simulink model "ame532Project1_GimbalDynamicsModel_2022b"  (R2022b)
settings: Solver=ode4  StartTime=0.0  StopTime=10  FixedStep=0.01  RelTol=1e-3
model workspace (MAT data in the model file):
  theta : Simulink.Parameter (value not decoded)
values from neighbouring files (symbols this model uses):
  a0_s2 = 0    [AeroData.m]
  a0_s3 = 0    [AeroData.m]
  a0_s4 = 0.05    [AeroData.m]
  a0_s5 = 0.05    [AeroData.m]
  CD0_s2 = 0.01    [AeroData.m]
  CD0_s3 = 0.01    [AeroData.m]
  CD0_s4 = 0.01    [AeroData.m]
  CD0_s5 = 0.01    [AeroData.m]
  CDa_s2 = 1    [AeroData.m]
  CDa_s3 = 1    [AeroData.m]
  CDa_s4 = 1    [AeroData.m]
  CDa_s5 = 1    [AeroData.m]
  CL0_s2 = 0    [AeroData.m]
  CL0_s3 = 0    [AeroData.m]
  CL0_s4 = 0.05    [AeroData.m]
  CL0_s5 = 0.05    [AeroData.m]
  CM0_s2 = 0    [AeroData.m]
  CM0_s3 = 0    [AeroData.m]
  CM0_s4 = -0.05    [AeroData.m]
  CM0_s5 = -0.05    [AeroData.m]
  CMa_s2 = 0    [AeroData.m]
  CMa_s3 = 0    [AeroData.m]
  CMa_s4 = 0    [AeroData.m]
  CMa_s5 = 0    [AeroData.m]
  e_s2 = 0.8    [AeroData.m]
  e_s3 = 0.8    [AeroData.m]
  e_s4 = 0.9    [AeroData.m]
  e_s5 = 0.9    [AeroData.m]
  i_s2 = 0    [AeroData.m]
  i_s3 = 0    [AeroData.m]
  i_s4 = 0.05    [AeroData.m]
  i_s5 = 0.05    [AeroData.m]
  Jxx = 1    [Sim_sixDOFdriverScript.m]
  Jxy = 0.    (= 0)    [Sim_sixDOFdriverScript.m]
  Jxz = 3    [Sim_sixDOFdriverScript.m]
  Jyx = 2    [Sim_sixDOFdriverScript.m]
  Jyy = 2    [Sim_sixDOFdriverScript.m]
  Jyz = 0    [Sim_sixDOFdriverScript.m]
  Jzx = Jxz    (= 3)    [Sim_sixDOFdriverScript.m]
  Jzy = Jyz    (= 0)    [Sim_sixDOFdriverScript.m]
  Jzz = 2    [Sim_sixDOFdriverScript.m]
  LL = 0.8    [Sim_sixDOFdriverScript.m]
  MM = 0.8    [Sim_sixDOFdriverScript.m]
  n_s2 = [0; 0; -1]    [AeroData.m]
  n_s3 = [0; 1; 0]    [AeroData.m]
  n_s4 = [0; 0; -1]    [AeroData.m]
  n_s5 = [0; 0; -1]    [AeroData.m]
  NN = 0.8    [Sim_sixDOFdriverScript.m]
  rEarth = 6378100    [Sim_sixDOFdriverScript.m]
  ro = 1.225    [AeroData.m]
undefined symbols (not defined in the file or in its folder): AR_s2, AR_s3, AR_s4, AR_s5, area_s2, area_s3, area_s4, area_s5, c_s2, c_s3, c_s4, c_s5, earthRadius, elevator_sA, leftaileron_sA, mixMatrixInv, rightaileron_sA, rudder_sA, totMass, x_S2_B_B, x_S3_B_B, x_S4_B_B, x_S5_B_B
libraries: simulink_extras x35, matrix_library x22, aerolibutil x8, aerolibfltsims x4, vrlib x4, aerolibtransform2 x2, sharedtransform x2, simulink x2, slpidlib x1, sharedutil x1
(part 3 of 5)

== system ame532Project1_GimbalDynamicsModel_2022b/Subsystem/Equations of Motion/TransKin_RotKin_TansDynam ==
  wBodyRates_PQR : Inport
  Aero Forces : Inport  Port=2
  InputV_B_E_B : Inport  Port=3
  LAX Initial Location : Inport  Port=4
  Constant : Constant  Value=[150 0 0]
  Manual Switch : ManualSwitch  CurrentSetting=0
  Mux2 : Mux  Inputs=3
  Pitch2_rad : Constant  Value=0
  Roll2_rad : Constant  Value=0
  Rotational Kinematics_Euler : Subsystem
  Rotational Kinematics_Quaternions : Subsystem
  Scope : Scope
  Translational Dynamics : Subsystem
  Translational Kinematics : Subsystem
  Yaw2_rad : Constant  Value=0
  Altitude_m : Outport
  C_B_N : Outport  Port=2
  OutputAccel_B_E_B : Outport  Port=3
  E_x_B_E_E : Outport  Port=4
  DCM C_EB : Outport  Port=5
  pos in LAX NED : Outport  Port=6
  wires:
  Pitch2_rad/1 -> Mux2/2
  wBodyRates_PQR/1 -> Translational Dynamics/2(wBodyRates_PQR), Rotational Kinematics_Quaternions/1(wVectorBodyRates_PQR), Rotational Kinematics_Euler/1(wVectorBodyRates_PQR)
  Roll2_rad/1 -> Mux2/1
  Yaw2_rad/1 -> Mux2/3
  Aero Forces/1 -> Translational Dynamics/3(Aero Forces)
  Mux2/1 -> Translational Kinematics/1(Custom Attitude w.r.t ECEF)  "User Defined Attitude w.r.t ECEF"
  Rotational Kinematics_Euler/1(Theta Vector_rad) -> Manual Switch/2  "Computed Attitude w.r.t ECEF"
  Constant/1 -> Translational Kinematics/3(Custom Body Lin Vel w.r.t ECEF)  "Custom Body Lin Vel w.r.t. ECEF"
  Translational Kinematics/1(Altitude_m) -> Altitude_m/1  "Altitude"
  Translational Kinematics/3(C_B_N) -> Translational Dynamics/1(C_B_N), C_B_N/1  "DCM from NED to Body"
  Translational Dynamics/1(Out_Vdot_B_E_B) -> OutputAccel_B_E_B/1  "Vdot_B_E_B  Acceleration of Body w.r.t ECEF measured in Body"
  InputV_B_E_B/1 -> Translational Dynamics/4(V_B_E_B), Translational Kinematics/4(Computed V_B_E_B)  "V_B_E_B  Velocity of Body w.r.t ECEF measured in Body"
  Translational Kinematics/2(E_x_B_E_E) -> E_x_B_E_E/1  "Position of Body w.r.t ECEF Measured in ECEF"
  Rotational Kinematics_Quaternions/1(Theta Vector_rad) -> Manual Switch/1
  Manual Switch/1 -> Scope/1, Translational Kinematics/2(Computed Attitude w.r.t ECEF)
  LAX Initial Location/1 -> Translational Kinematics/5(LAX Initial Location)
  Translational Kinematics/4(DCM C_EB) -> DCM C_EB/1
  Translational Kinematics/5(position in LAX NED) -> pos in LAX NED/1

== system ame532Project1_GimbalDynamicsModel_2022b/Subsystem/IMU/Accelerometer ==
  True Acceleration : Inport
  Band-Limited White Noise : simulink/Sources/Band-Limited White Noise  Cov=[0.000001]  Ts=0.1  seed=[23341]
  Bias : Constant  Value=[0.025*9.8 0.025*9.8 0.025*9.8]
  Scale Factor : Gain  Gain=0.001
  Sum : Sum  Inputs=|++
  Sum1 : Sum  Inputs=|++
  Measured Acceleration : Outport
  wires:
  True Acceleration/1 -> Sum/1
  Bias/1 -> Sum/2
  Sum/1 -> Scale Factor/1
  Scale Factor/1 -> Sum1/1
  Band-Limited White Noise/1 -> Sum1/2
  Sum1/1 -> Measured Acceleration/1

== system ame532Project1_GimbalDynamicsModel_2022b/Subsystem/IMU/Gyroscope ==
  True Body Rates : Inport
  Band-Limited White Noise : simulink/Sources/Band-Limited White Noise  Commented=on  Cov=[0.000001]  Ts=0.1  seed=[23341]
  Gyro Constant Bias : Constant  Value=[0.025*9.8 0.025*9.8 0.025*9.8]
  Gyro Scale Factor : Gain  Gain=0.001
  Sum : Sum  Inputs=|++
  Sum1 : Sum  Inputs=|++
  Measured Body Rates : Outport
  wires:
  True Body Rates/1 -> Sum/1
  Gyro Constant Bias/1 -> Sum/2
  Sum/1 -> Gyro Scale Factor/1
  Gyro Scale Factor/1 -> Sum1/1
  Band-Limited White Noise/1 -> Sum1/2
  Sum1/1 -> Measured Body Rates/1

== system ame532Project1_GimbalDynamicsModel_2022b/Subsystem/Equations of Motion/Aero Forces and Moments/F&M Horiz Stab Surface (S2) ==
  v_B_E_B : Inport
  V_B_A_B (Relative AIr Speed) : Inport  Port=2
  ElevatorControl : Inport  Port=3
  Compute Aero Lift and Drag : MATLAB Function  TreatAsAtomicUnit=on
  Compute Aero Moment : MATLAB Function  TreatAsAtomicUnit=on
  Constant : Constant  Value=[AR_s2 i_s2 CL0_s2 CD0_s2 CDa_s2 a0_s2 e_s2 ro area_s2 elevator_sA]
  Constant1 : Constant  Value=[CM0_s2; CMa_s2; c_s2]
  Demux : Demux  Outputs=10
  Demux1 : Demux  Outputs=3
  F&M in Body : Subsystem
  n_s2 : Constant  Value=n_s2
  momS2_B : Outport
  LiftAndDragForceS2_B : Outport  Port=2
  wires:
  Compute Aero Lift and Drag/2(liftSurf) -> F&M in Body/2(Lift)  "Lift Force w.r.t Wind"
  Compute Aero Moment/1(momSurf) -> F&M in Body/1(momSurf)  "Moment of Surface w.r.t Wind"
  Compute Aero Lift and Drag/3(dragSurf) -> F&M in Body/3(Drag)  "Drag Force w.r.t Wind"
  F&M in Body/2(LiftAndDragForceS2_B) -> LiftAndDragForceS2_B/1
  Compute Aero Lift and Drag/1(alphaLocal) -> Compute Aero Moment/2(alphaLocal)
  F&M in Body/1(momS2_B) -> momS2_B/1
  V_B_A_B (Relative AIr Speed)/1 -> Compute Aero Lift and Drag/1(v_B_A_B), F&M in Body/4(v_B_A_B)
  Constant/1 -> Demux/1
  Demux/1 -> Compute Aero Lift and Drag/2(AR_s2)  "AR_s2"
  Demux/2 -> Compute Aero Lift and Drag/3(i_s2)  "i_s2"
  Demux/3 -> Compute Aero Lift and Drag/5(CL0_s2)  "CL0_s2"
  Demux/4 -> Compute Aero Lift and Drag/6(CD0_s2)  "CD0_s2"
  Demux/5 -> Compute Aero Lift and Drag/7(CDa_s2)  "CDa_s2"
  Demux/6 -> Compute Aero Lift and Drag/8(a0_s2)  "a0_s2"
  Demux/7 -> Compute Aero Lift and Drag/9(e_s2)  "e_s2"
  Demux/8 -> Compute Aero Moment/5(ro), Compute Aero Lift and Drag/10(ro)  "ro"
  Demux/9 -> Compute Aero Moment/6(area_s2), Compute Aero Lift and Drag/11(area_s2)  "area_s2"
  Constant1/1 -> Demux1/1
  Demux1/1 -> Compute Aero Moment/3(CM0_s2)  "CMo_s2"
  Demux1/2 -> Compute Aero Moment/4(CMa_s2)  "CMa_s2"
  Demux1/3 -> Compute Aero Moment/7(c_s2)  "c_s2"
  n_s2/1 -> F&M in Body/5(n_s2), Compute Aero Lift and Drag/4(n_s2)
  ElevatorControl/1 -> Compute Aero Lift and Drag/12(elevatorControl)
  Demux/10 -> Compute Aero Lift and Drag/13(elevatorArea_uControl)
  v_B_E_B/1 -> Compute Aero Moment/1(V_B_A_B)

== system ame532Project1_GimbalDynamicsModel_2022b/Subsystem/Equations of Motion/Aero Forces and Moments/F&M Horiz Stab Surface (S3) ==
  v_B_E_B : Inport
  V_B_A_B (Relative AIr Speed) : Inport  Port=2
  RudderControl : Inport  Port=3
  Compute Aero Lift and Drag : MATLAB Function  TreatAsAtomicUnit=on
  Compute Aero Moment : MATLAB Function  TreatAsAtomicUnit=on
  Constant : Constant  Value=[AR_s3 i_s3 CL0_s3 CD0_s3 CDa_s3 a0_s3 e_s3 ro area_s3 rudder_sA]
  Constant1 : Constant  Value=[CM0_s3; CMa_s3; c_s3]
  Constant2 : Constant  Value=n_s3
  Demux : Demux  Outputs=10
  Demux1 : Demux  Outputs=3
  F&M in Body : Subsystem
  momS3_B : Outport
  LiftAndDragForceS3_B : Outport  Port=2
  wires:
  Compute Aero Lift and Drag/2(liftSurf) -> F&M in Body/2(Lift)  "Lift Force w.r.t Wind"
  Compute Aero Moment/1(momSurf) -> F&M in Body/1(momSurf)  "Moment of Surface w.r.t Wind"
  Compute Aero Lift and Drag/3(dragSurf) -> F&M in Body/3(Drag)  "Drag Force w.r.t Wind"
  F&M in Body/2(LiftAndDragForceS3_B) -> LiftAndDragForceS3_B/1
  Compute Aero Lift and Drag/1(alphaLocal) -> Compute Aero Moment/2(alphaLocal)
  F&M in Body/1(momS3_B) -> momS3_B/1
  V_B_A_B (Relative AIr Speed)/1 -> F&M in Body/4(v_B_A_B), Compute Aero Lift and Drag/1(v_B_A_B)
  Constant/1 -> Demux/1
  Demux/1 -> Compute Aero Lift and Drag/2(AR_s3)  "AR_s3"
  Demux/2 -> Compute Aero Lift and Drag/3(i_s3)  "i_s3"
  Constant2/1 -> F&M in Body/5(n_s3), Compute Aero Lift and Drag/4(n_s3)  "n_s3"
  Demux/3 -> Compute Aero Lift and Drag/5(CL0_s3)  "CL0_s3"
  Demux/4 -> Compute Aero Lift and Drag/6(CD0_s3)  "CD0_s3"
  Demux/5 -> Compute Aero Lift and Drag/7(CDa_s3)  "CDa_s3"
  Demux/6 -> Compute Aero Lift and Drag/8(a0_s3)  "a0_s3"
  Demux/7 -> Compute Aero Lift and Drag/9(e_s3)  "e_s3"
  Demux/8 -> Compute Aero Moment/5(ro), Compute Aero Lift and Drag/10(ro)  "ro"
  Demux/9 -> Compute Aero Moment/6(area_s3), Compute Aero Lift and Drag/11(area_s3)  "area_s3"
  Constant1/1 -> Demux1/1
  Demux1/1 -> Compute Aero Moment/3(CM0_s3)  "CMo_s3"
  Demux1/2 -> Compute Aero Moment/4(CMa_s3)  "CMa_s3"
  Demux1/3 -> Compute Aero Moment/7(c_s3)  "c_s3"
  RudderControl/1 -> Compute Aero Lift and Drag/12(rudderControl)
  Demux/10 -> Compute Aero Lift and Drag/13(rudderarea_uControl)
  v_B_E_B/1 -> Compute Aero Moment/1(V_B_A_B)

== system ame532Project1_GimbalDynamicsModel_2022b/Subsystem/Equations of Motion/Aero Forces and Moments/F&M Right Wing and Servo Surface (S4) ==
  v_B_E_B : Inport
  V_B_A_B (Relative AIr Speed) : Inport  Port=2
  RightAileronControl : Inport  Port=3
  Compute Aero Lift and Drag : MATLAB Function  TreatAsAtomicUnit=on
  Compute Aero Moment : MATLAB Function  TreatAsAtomicUnit=on
  Constant : Constant  Value="[AR_s4 i_s4  CL0_s4 CD0_s4 CDa_s4 a0_s4 e_s4 ro area_s4 rightaileron_sA]"
  Constant1 : Constant  Value=[CM0_s4; CMa_s4; c_s4]
  Demux : Demux  Outputs=10
  Demux1 : Demux  Outputs=3
  F&M in Body : Subsystem
  n_s4 : Constant  Value=n_s4
  momS4_B : Outport
  LiftAndDragForceS4_B : Outport  Port=2
  wires:
  Compute Aero Lift and Drag/2(liftSurf) -> F&M in Body/2(Lift)  "Lift Force w.r.t Wind"
  Compute Aero Moment/1(momSurf) -> F&M in Body/1(momSurf)  "Moment of Surface w.r.t Wind"
  Compute Aero Lift and Drag/3(dragSurf) -> F&M in Body/3(Drag)  "Drag Force w.r.t Wind"
  F&M in Body/2(LiftAndDragForceS4_B) -> LiftAndDragForceS4_B/1
  Compute Aero Lift and Drag/1(alphaLocal) -> Compute Aero Moment/2(alphaLocal)
  F&M in Body/1(momS4_B) -> momS4_B/1
  V_B_A_B (Relative AIr Speed)/1 -> F&M in Body/4(v_B_A_B), Compute Aero Lift and Drag/1(v_B_A_B)
  Constant/1 -> Demux/1
  Demux/1 -> Compute Aero Lift and Drag/2(AR_s4)  "AR_s4"
  Demux/2 -> Compute Aero Lift and Drag/3(i_s4)  "i_s4"
  n_s4/1 -> F&M in Body/5(n_s4), Compute Aero Lift and Drag/4(n_s4)  "n_s4"
  Demux/3 -> Compute Aero Lift and Drag/5(CL0_s4)  "CL0_s4"
  Demux/4 -> Compute Aero Lift and Drag/6(CD0_s4)  "CD0_s4"
  Demux/5 -> Compute Aero Lift and Drag/7(CDa_s4)  "CDa_s4"
  Demux/6 -> Compute Aero Lift and Drag/8(a0_s4)  "a0_s4"
  Demux/7 -> Compute Aero Lift and Drag/9(e_s4)  "e_s4"
  Demux/9 -> Compute Aero Moment/6(area_s4), Compute Aero Lift and Drag/11(area_s4)  "area_s4"
  Constant1/1 -> Demux1/1
  Demux1/1 -> Compute Aero Moment/3(CM0_s4)  "CMo_s4"
  Demux1/2 -> Compute Aero Moment/4(CMa_s4)  "CMa_s4"
  Demux1/3 -> Compute Aero Moment/7(c_s4)  "c_s4"
  Demux/8 -> Compute Aero Moment/5(ro), Compute Aero Lift and Drag/10(ro)  "e_s4"
  RightAileronControl/1 -> Compute Aero Lift and Drag/12(rightAileronControl)
  Demux/10 -> Compute Aero Lift and Drag/13(rightaileronArea_uControl)
  v_B_E_B/1 -> Compute Aero Moment/1(V_B_A_B)

== system ame532Project1_GimbalDynamicsModel_2022b/Subsystem/Equations of Motion/Aero Forces and Moments/F&M Right Wing and Servo Surface (S5) ==
  v_B_E_B : Inport
  V_B_A_B (Relative AIr Speed) : Inport  Port=2
  LeftAileronControl : Inport  Port=3
  Compute Aero Lift and Drag : MATLAB Function  TreatAsAtomicUnit=on
  Compute Aero Moment : MATLAB Function  TreatAsAtomicUnit=on
  Constant : Constant  Value=[AR_s5 i_s5 CL0_s5 CD0_s5 CDa_s5 a0_s5 e_s5 ro area_s5 leftaileron_sA]
  Constant1 : Constant  Value=[CM0_s5; CMa_s5; c_s5]
  Demux : Demux  Outputs=10
  Demux1 : Demux  Outputs=3
  F&M in Body : Subsystem
  n_s5 : Constant  Value=n_s5
  momS5_B : Outport
  LiftAndDragForceS5_B : Outport  Port=2
  wires:
  Compute Aero Lift and Drag/2(liftSurf) -> F&M in Body/2(Lift)  "Lift Force w.r.t Wind"
  Compute Aero Moment/1(momSurf) -> F&M in Body/1(momSurf)  "Moment of Surface w.r.t Wind"
  Compute Aero Lift and Drag/3(dragSurf) -> F&M in Body/3(Drag)  "Drag Force w.r.t Wind"
  F&M in Body/2(LiftAndDragForceS5_B) -> LiftAndDragForceS5_B/1
  Compute Aero Lift and Drag/1(alphaLocal) -> Compute Aero Moment/2(alphaLocal)
  F&M in Body/1(momS5_B) -> momS5_B/1
  V_B_A_B (Relative AIr Speed)/1 -> F&M in Body/4(v_B_A_B), Compute Aero Lift and Drag/1(v_B_A_B)
  Constant/1 -> Demux/1
  Demux/1 -> Compute Aero Lift and Drag/2(AR_s5)  "AR_s5"
  Demux/2 -> Compute Aero Lift and Drag/3(i_s5)  "i_s5"
  n_s5/1 -> Compute Aero Lift and Drag/4(n_s5), F&M in Body/5(n_s5)  "n_s5"
  Demux/3 -> Compute Aero Lift and Drag/5(CL0_s5)  "CL0_s5"
  Demux/4 -> Compute Aero Lift and Drag/6(CD0_s5)  "CD0_s5"
  Demux/5 -> Compute Aero Lift and Drag/7(CDa_s5)  "CDa_s5"
  Demux/6 -> Compute Aero Lift and Drag/8(a0_s5)  "a0_s5"
  Demux/7 -> Compute Aero Lift and Drag/9(e_s5)  "e_s5"
  Demux/8 -> Compute Aero Moment/5(ro), Compute Aero Lift and Drag/10(ro)  "ro"
  Demux/9 -> Compute Aero Moment/6(area_s5), Compute Aero Lift and Drag/11(area_s5)  "area_s5"
  Constant1/1 -> Demux1/1
  Demux1/1 -> Compute Aero Moment/3(CM0_s5)  "CMo_s5"
  Demux1/2 -> Compute Aero Moment/4(CMa_s5)  "CMa_s5"
  Demux1/3 -> Compute Aero Moment/7(c_s5)  "c_s5"
  LeftAileronControl/1 -> Compute Aero Lift and Drag/12(leftAileronControl)
  Demux/10 -> Compute Aero Lift and Drag/13(leftAileronArea_uControl)
  v_B_E_B/1 -> Compute Aero Moment/1(V_B_A_B)

== system ame532Project1_GimbalDynamicsModel_2022b/Subsystem/Equations of Motion/Rotational Dynamics/Using Cross Product Matrix ==
  wPQR : Inport
  J Matrix : Inport  Port=2
  Matrix Multiply : Product  Multiplication=Matrix(*)
  Matrix Multiply1 : Product  Multiplication=Matrix(*)
  Omega Cross Matrix : MATLAB Function  TreatAsAtomicUnit=on
  OmegaJw : Outport
  wires:
  wPQR/1 -> Omega Cross Matrix/1(PQR), Matrix Multiply1/2
  J Matrix/1 -> Matrix Multiply1/1
  Omega Cross Matrix/1(omegaMat) -> Matrix Multiply/1
  Matrix Multiply1/1 -> Matrix Multiply/2  "Jw"
  Matrix Multiply/1 -> OmegaJw/1

== system ame532Project1_GimbalDynamicsModel_2022b/Subsystem/Equations of Motion/Rotational Dynamics/Using Cross Product Operator Only ==
  wPQR : Inport
  J Matrix : Inport  Port=2
  Cross Product : matrix_library/Cross Product
  Matrix Multiply1 : Product  Multiplication=Matrix(*)
  OmegaJw : Outport
  wires:
  wPQR/1 -> Matrix Multiply1/2, Cross Product/1
  J Matrix/1 -> Matrix Multiply1/1
  Matrix Multiply1/1 -> Cross Product/2  "Jw"
  Cross Product/1 -> OmegaJw/1

== system ame532Project1_GimbalDynamicsModel_2022b/Subsystem/Equations of Motion/TransKin_RotKin_TansDynam/Rotational Kinematics_Euler ==
  wVectorBodyRates_PQR : Inport
  Demux : Demux  Outputs=3
  EulerAngles : Integrator  InitialConditionSource=external  InitialCondition=[0;30;30]  ContinuousStateAttributes='EulerAngles_PhiThetaPsi'
  HinvMatrix : MATLAB Function  TreatAsAtomicUnit=on
  Initial Attitude_rad w.r.t ECEF : Constant  Value=[0; 0; 0]
  MatrixMultiply : Product  Multiplication=Matrix(*)
  Scope : Scope
  Terminator : Terminator
  Theta Vector_rad : Outport
  wires:
  HinvMatrix/1(hinv) -> MatrixMultiply/1
  MatrixMultiply/1 -> EulerAngles/1  "Theta Vector Dot"
  EulerAngles/1 -> Demux/1, Theta Vector_rad/1, Scope/1  "Theta Vector_rad"
  Demux/1 -> HinvMatrix/2(rollPhi)  "roll_rad"
  Demux/2 -> HinvMatrix/1(pitchTheta)  "pitch_rad"
  Demux/3 -> Terminator/1  "yaw_rad"
  wVectorBodyRates_PQR/1 -> MatrixMultiply/2  "wVector Body Rates_PQR"
  Initial Attitude_rad w.r.t ECEF/1 -> EulerAngles/2

== system ame532Project1_GimbalDynamicsModel_2022b/Subsystem/Equations of Motion/TransKin_RotKin_TansDynam/Rotational Kinematics_Quaternions ==
  wVectorBodyRates_PQR : Inport
  Constant : Constant  Value=0
  Degrees to Radians : simulink_extras/Transformations/Degrees to Radians
  Gain : Gain  Gain=0.5
  Initial Attitude_rad w.r.t ECEF : Constant  Value=[0; 0; 0]
  Integrator : Integrator  InitialConditionSource=external
  Manual Switch : ManualSwitch  CurrentSetting=0
  Mux : Mux  Inputs=3
  Normalize Vector : vrlib/Utilities/Normalize Vector  maxzero=0
  NormalizeQuaternion : MATLAB Function  Commented=on  TreatAsAtomicUnit=on
  Quaternion Multiplication : aerolibutil/Quaternion Multiplication
  Quaternions to Rotation Angles : sharedtransform/Quaternions to Rotation Angles  rotationOrder=ZYX  aMode=aMode
  Rotation Angles to Quaternions : sharedtransform/Rotation Angles to Quaternions  rotationOrder=ZYX  aMode=aMode
  Vector Concatenate : Concatenate
  quaternionMultiplication : MATLAB Function  Commented=on  TreatAsAtomicUnit=on
  quaternionToeuler : MATLAB Function  TreatAsAtomicUnit=on
  Theta Vector_rad : Outport
  wires:
  wVectorBodyRates_PQR/1 -> Gain/1
  Gain/1 -> Vector Concatenate/2
  Constant/1 -> Vector Concatenate/1
  quaternionToeuler/3(roll_deg) -> Mux/1
  quaternionToeuler/2(pitch_deg) -> Mux/2
  quaternionToeuler/1(yaw_deg) -> Mux/3
  Mux/1 -> Manual Switch/1
  Quaternion Multiplication/1 -> Integrator/1
  Vector Concatenate/1 -> Quaternion Multiplication/2
  Initial Attitude_rad w.r.t ECEF/1 -> Degrees to Radians/1
  Degrees to Radians/1 -> Rotation Angles to Quaternions/1
  Rotation Angles to Quaternions/1 -> Integrator/2
  Normalize Vector/1 -> Quaternion Multiplication/1, Quaternions to Rotation Angles/1, quaternionToeuler/1(qin)
  Quaternions to Rotation Angles/1 -> Manual Switch/2
  Manual Switch/1 -> Theta Vector_rad/1
  Integrator/1 -> Normalize Vector/1  "q_B_N"

== system ame532Project1_GimbalDynamicsModel_2022b/Subsystem/Equations of Motion/TransKin_RotKin_TansDynam/Translational Dynamics ==
  C_B_N : Inport
  wBodyRates_PQR : Inport  Port=2
  Aero Forces : Inport  Port=3
  V_B_E_B : Inport  Port=4
  Constant : Constant  Value=totMass
  Cross Product : matrix_library/Cross Product
  Display : Display
  Divide : Product  Inputs=*/
  Gravity in N Frame : Constant  Value=[0 0 9.81]
  Matrix Multiply : Product  Multiplication=Matrix(*)
  Sum : Sum  Inputs=|++-
  Out_Vdot_B_E_B : Outport
  wires:
  wBodyRates_PQR/1 -> Cross Product/1
  Cross Product/1 -> Sum/3  "Vdot_B_E_B"
  Sum/1 -> Out_Vdot_B_E_B/1  "True Vdot_B_E_B"
  Gravity in N Frame/1 -> Matrix Multiply/2
  C_B_N/1 -> Matrix Multiply/1  "c_B_N"
  Matrix Multiply/1 -> Sum/2
  Aero Forces/1 -> Divide/1
  V_B_E_B/1 -> Cross Product/2
  Constant/1 -> Display/1, Divide/2
  Divide/1 -> Sum/1

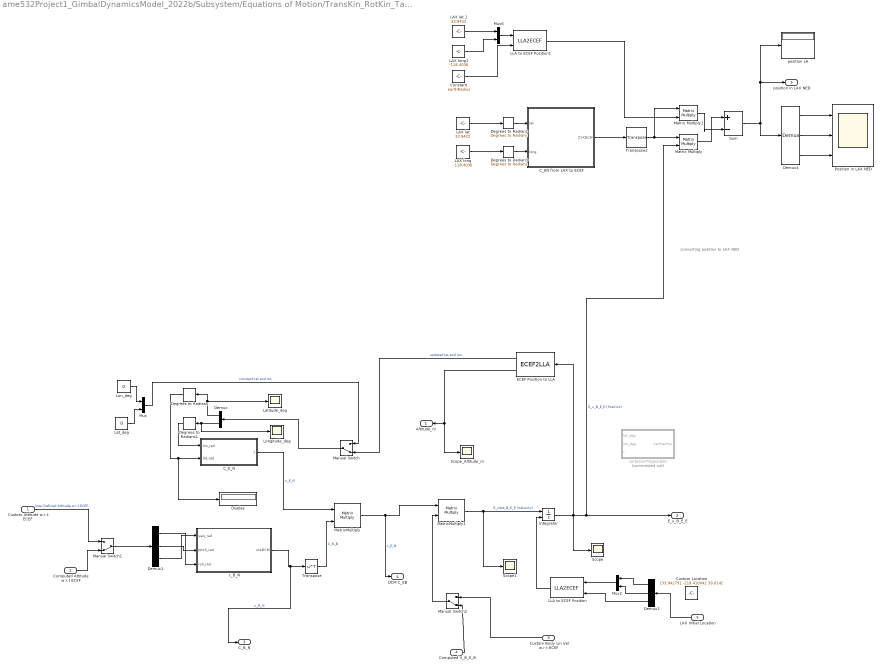
== system ame532Project1_GimbalDynamicsModel_2022b/Subsystem/Equations of Motion/TransKin_RotKin_TansDynam/Translational Kinematics ==
  note: converting position to LAX NED
  Custom Attitude w.r.t ECEF : Inport
  Computed Attitude w.r.t ECEF : Inport  Port=2
  Custom Body Lin Vel w.r.t ECEF : Inport  Port=3
  Computed V_B_E_B : Inport  Port=4
  LAX Initial Location : Inport  Port=5
  C_EN from LAX to ECEF : MATLAB Function  TreatAsAtomicUnit=on
  C_E_N : MATLAB Function  TreatAsAtomicUnit=on
  Constant : Constant  Value=earthRadius
  Custom Location : Constant  Value=[33.942791 -118.410042 39.014]'
  Degrees to Radian2 : simulink_extras/Transformations/Degrees to Radians
  Degrees to Radian3 : simulink_extras/Transformations/Degrees to Radians
  Degrees to Radians : simulink_extras/Transformations/Degrees to Radians
  Degrees to Radians1 : simulink_extras/Transformations/Degrees to Radians
  Demux : Demux  Outputs=2
  Demux1 : Demux  Outputs=3
  Demux2 : Demux  Outputs=3
  Demux4 : Demux  Outputs=3
  Display : Display
  ECEF Position to LLA : ECEF2LLA  ptype=Custom
  Integrator : Integrator  InitialConditionSource=external  InitialCondition=[0;0;rEarth]  ContinuousStateAttributes='Position'
  "LAX lat " : Constant  Value=33.9422
  LAX lat 1 : Constant  Value=33.9422
  LAX long : Constant  Value=-118.4036
  LAX long1 : Constant  Value=-118.4036
  LLA to ECEF Position : LLA2ECEF  ptype=Custom
  LLA to ECEF Position1 : LLA2ECEF
  Lat_deg : Constant  Value=0
  Latitude_deg : Scope
  Lon_deg : Constant  Value=0
  Longitude_deg : Scope
  Manual Switch : ManualSwitch  CurrentSetting=0
  Manual Switch1 : ManualSwitch  CurrentSetting=0
  Manual Switch2 : ManualSwitch  CurrentSetting=0
  Matrix Multiply : Product  Multiplication=Matrix(*)
  Matrix Multiply1 : Product  Multiplication=Matrix(*)
  MatrixMultiply : Product  Multiplication=Matrix(*)
  MatrixMultiply1 : Product  Multiplication=Matrix(*)
  Mux : Mux  Inputs=2
  Mux2 : Mux  Inputs=2
  Mux6 : Mux  Inputs=2
  Position in LAX NED : Scope  NumInputPorts=3
  Scope : Scope
  Scope1 : Scope
  Scope_Altitude_m : Scope
  Sum : Sum  Inputs=|+-
  Transpose : Math  Operator=transpose
  Transpose2 : matrix_library/Transpose
  c_B_N : MATLAB Function  TreatAsAtomicUnit=on
  cartesianTOgeodetic : MATLAB Function  Commented=on  TreatAsAtomicUnit=on
  "position LA " : Display
  Altitude_m : Outport
  E_x_B_E_E : Outport  Port=2
  C_B_N : Outport  Port=3
  DCM C_EB : Outport  Port=4
  position in LAX NED : Outport  Port=5
  wires:
  MatrixMultiply1/1 -> Scope1/1, Integrator/1  "E_xdot_B_E_E (Velocity)"
  C_E_N/1(y) -> MatrixMultiply/1  "c_E_N"
  Manual Switch1/1 -> Demux1/1
  MatrixMultiply/1 -> DCM C_EB/1, MatrixMultiply1/1  "c_E_B"
  Degrees to Radians/1 -> Display/1, C_E_N/2(lat_rad)
  ECEF Position to LLA/2 -> Altitude_m/1, Scope_Altitude_m/1
  Transpose/1 -> MatrixMultiply/2  "C_N_B"
  Lon_deg/1 -> Mux/1
  Mux/1 -> Manual Switch/1  "constant lat and lon"
  Lat_deg/1 -> Mux/2
  Integrator/1 -> ECEF Position to LLA/1, Matrix Multiply/2, E_x_B_E_E/1, Scope/1  "E_x_B_E_E (Position)"
  ECEF Position to LLA/1 -> Manual Switch/2  "updated lat and lon"
  Demux1/3 -> c_B_N/1(yaw_rad)
  Demux1/1 -> c_B_N/3(roll_rad)
  Demux1/2 -> c_B_N/2(pitch_rad)
  c_B_N/1(outDCM) -> C_B_N/1, Transpose/1  "c_B_N"
  Manual Switch/1 -> Demux/1
  Manual Switch2/1 -> MatrixMultiply1/2
  Custom Attitude w.r.t ECEF/1 -> Manual Switch1/1  "User Defined Attitude w.r.t ECEF"
  Computed Attitude w.r.t ECEF/1 -> Manual Switch1/2
  Custom Body Lin Vel w.r.t ECEF/1 -> Manual Switch2/1
  Computed V_B_E_B/1 -> Manual Switch2/2
  Demux/2 -> Longitude_deg/1, Degrees to Radians1/1
  Demux/1 -> Degrees to Radians/1, Latitude_deg/1
  Degrees to Radians1/1 -> C_E_N/1(lon_rad)
  Demux2/1 -> Mux2/1
  Demux2/2 -> Mux2/2
  Demux2/3 -> LLA to ECEF Position/2
  Mux2/1 -> LLA to ECEF Position/1
  LLA to ECEF Position/1 -> Integrator/2
  LAX Initial Location/1 -> Demux2/1
  Demux4/1 -> Position in LAX NED/1
  Transpose2/1 -> Matrix Multiply1/1, Matrix Multiply/1
  "LAX lat "/1 -> Degrees to Radian2/1
  Matrix Multiply1/1 -> Sum/2
  C_EN from LAX to ECEF/1(ZYXDCM) -> Transpose2/1
  Demux4/3 -> Position in LAX NED/3
  LLA to ECEF Position1/1 -> Matrix Multiply1/2
  Matrix Multiply/1 -> Sum/1
  Constant/1 -> LLA to ECEF Position1/2
  Sum/1 -> "position LA "/1, position in LAX NED/1, Demux4/1
  Degrees to Radian2/1 -> C_EN from LAX to ECEF/1(lat)
  Demux4/2 -> Position in LAX NED/2
  LAX long1/1 -> Mux6/2
  Degrees to Radian3/1 -> C_EN from LAX to ECEF/2(long)
  Mux6/1 -> LLA to ECEF Position1/1
  LAX long/1 -> Degrees to Radian3/1
  LAX lat 1/1 -> Mux6/1

== system ame532Project1_GimbalDynamicsModel_2022b/Subsystem/Equations of Motion/Aero Forces and Moments/F&M Horiz Stab Surface (S2)/F&M in Body ==
  momSurf : Inport
  Lift : Inport  Port=2
  Drag : Inport  Port=3
  v_B_A_B : Inport  Port=4
  n_s2 : Inport  Port=5
  Constant : Constant  Value=x_S2_B_B
  Force Due to Lift and Drag : MATLAB Function  TreatAsAtomicUnit=on
  Moment S2 : MATLAB Function  TreatAsAtomicUnit=on
  momS2_B : Outport
  LiftAndDragForceS2_B : Outport  Port=2
  wires:
  momSurf/1 -> Moment S2/1(momSurf)
  Lift/1 -> Force Due to Lift and Drag/1(lift)
  Drag/1 -> Force Due to Lift and Drag/2(drag)
  Force Due to Lift and Drag/1(forceLiftDragS2_B) -> Moment S2/2(FliftdragS), LiftAndDragForceS2_B/1
  v_B_A_B/1 -> Force Due to Lift and Drag/3(v_B_A_B)
  Moment S2/1(momS2_B) -> momS2_B/1
  n_s2/1 -> Force Due to Lift and Drag/4(n_s2), Moment S2/3(n_s2)
  Constant/1 -> Moment S2/4(x_S2_B_B)

== system ame532Project1_GimbalDynamicsModel_2022b/Subsystem/Equations of Motion/Aero Forces and Moments/F&M Horiz Stab Surface (S3)/F&M in Body ==
  momSurf : Inport
  Lift : Inport  Port=2
  Drag : Inport  Port=3
  v_B_A_B : Inport  Port=4
  n_s3 : Inport  Port=5
  Constant : Constant  Value=x_S3_B_B
  Force Due to Lift and Drag : MATLAB Function  TreatAsAtomicUnit=on
  Moment S3 : MATLAB Function  TreatAsAtomicUnit=on
  momS3_B : Outport
  LiftAndDragForceS3_B : Outport  Port=2
  wires:
  momSurf/1 -> Moment S3/1(momSurf)
  Lift/1 -> Force Due to Lift and Drag/1(lift)
  Drag/1 -> Force Due to Lift and Drag/2(drag)
  Force Due to Lift and Drag/1(forceLiftDragS3_B) -> Moment S3/2(FliftdragS), LiftAndDragForceS3_B/1
  v_B_A_B/1 -> Force Due to Lift and Drag/3(v_B_A_B)
  Moment S3/1(momS3_B) -> momS3_B/1
  n_s3/1 -> Force Due to Lift and Drag/4(n_s3), Moment S3/3(n_s3)
  Constant/1 -> Moment S3/4(x_S3_B_B)

== system ame532Project1_GimbalDynamicsModel_2022b/Subsystem/Equations of Motion/Aero Forces and Moments/F&M Right Wing and Servo Surface (S4)/F&M in Body ==
  momSurf : Inport
  Lift : Inport  Port=2
  Drag : Inport  Port=3
  v_B_A_B : Inport  Port=4
  n_s4 : Inport  Port=5
  Constant : Constant  Value=x_S4_B_B
  Force Due to Lift and Drag : MATLAB Function  TreatAsAtomicUnit=on
  Moment S4 : MATLAB Function  TreatAsAtomicUnit=on
  momS4_B : Outport
  LiftAndDragForceS4_B : Outport  Port=2
  wires:
  momSurf/1 -> Moment S4/1(momSurf)
  Lift/1 -> Force Due to Lift and Drag/1(lift)
  Drag/1 -> Force Due to Lift and Drag/2(drag)
  Force Due to Lift and Drag/1(forceLiftDragS4_B) -> Moment S4/2(FliftdragS), LiftAndDragForceS4_B/1
  v_B_A_B/1 -> Force Due to Lift and Drag/3(v_B_A_B)
  Moment S4/1(momS4_B) -> momS4_B/1
  n_s4/1 -> Force Due to Lift and Drag/4(n_s4), Moment S4/3(n_s4)
  Constant/1 -> Moment S4/4(x_S4_B_B)

== system ame532Project1_GimbalDynamicsModel_2022b/Subsystem/Equations of Motion/Aero Forces and Moments/F&M Right Wing and Servo Surface (S5)/F&M in Body ==
  momSurf : Inport
  Lift : Inport  Port=2
  Drag : Inport  Port=3
  v_B_A_B : Inport  Port=4
  n_s5 : Inport  Port=5
  Constant : Constant  Value=x_S5_B_B
  Force Due to Lift and Drag : MATLAB Function  TreatAsAtomicUnit=on
  Moment S5 : MATLAB Function  TreatAsAtomicUnit=on
  momS5_B : Outport
  LiftAndDragForceS5_B : Outport  Port=2
  wires:
  momSurf/1 -> Moment S5/1(momSurf)
  Lift/1 -> Force Due to Lift and Drag/1(lift)
  Drag/1 -> Force Due to Lift and Drag/2(drag)
  Force Due to Lift and Drag/1(forceLiftDragS5_B) -> Moment S5/2(FliftdragS), LiftAndDragForceS5_B/1
  v_B_A_B/1 -> Force Due to Lift and Drag/3(v_B_A_B)
  Moment S5/1(momS5_B) -> momS5_B/1
  n_s5/1 -> Force Due to Lift and Drag/4(n_s5), Moment S5/3(n_s5)
  Constant/1 -> Moment S5/4(x_S5_B_B)

== matlab function ame532Project1_GimbalDynamicsModel_2022b/Subsystem/Equations of Motion/Aero Forces and Moments/F&M Right Wing and Servo Surface (S5)/F&M in Body/Moment S5 ==
  data: momSurf input; momS5_B output; FliftdragS input; n_s5 input; x_S5_B_B input
function momS5_B = fcn(momSurf, FliftdragS, n_s5, x_S5_B_B)
% Compute the moment at the respective surface
crot = [0,0,0; 0,0,-1; 0,1,0];

momS5_B = momSurf * crot* n_s5 + (cross(x_S5_B_B, FliftdragS));

== matlab function ame532Project1_GimbalDynamicsModel_2022b/Subsystem/Equations of Motion/Rotational Dynamics/Using Cross Product Matrix/Omega Cross Matrix ==
  data: PQR input; omegaMat output
function omegaMat = fcn(PQR)
P = PQR(1); % deg
Q = PQR(2); % deg
R = PQR(3); % deg
omegaMat = [0 -R Q; R 0 -P; -Q P 0];

== matlab function ame532Project1_GimbalDynamicsModel_2022b/Gimbal Aircraft dynamic sim/Rotational Kinematics/C_EN2 ==
  data: roll input; ZYXDCM output; pitch input; yaw input
function ZYXDCM = DCM_from_Euler(roll,pitch,yaw) % sequence is yaw pitch roll
    yaw_matrix = [cos(yaw) -sin(yaw) 0;
                  sin(yaw) cos(yaw) 0;
                  0 0 1];
    pitch_matrix = [cos(pitch) 0 sin(pitch);
                    0           1           0;
                    -sin(pitch) 0  cos(pitch)];
    roll_matrix = [1            0           0;
                    0          cos(roll)    -sin(roll);
                    0           sin(roll)  cos(roll)];
    ZYXDCM = roll_matrix*pitch_matrix*yaw_matrix;
end

== matlab function ame532Project1_GimbalDynamicsModel_2022b/Subsystem/Equations of Motion/Rotational Kinematics_Quaternions/NormalizeQuaternion ==
  data: qin input; qoutNorm output
function qoutNorm = NormalizeQuaternion(qin)
qinMag = norm(qin);
qoutNorm = qin/qinMag;

== matlab function ame532Project1_GimbalDynamicsModel_2022b/Subsystem/Equations of Motion/Rotational Kinematics_Quaternions/quaternionMultiplication ==
  data: q1 input; qResult output; q2 input
function qResult = quaternionMultiplication(q1,q2)
q1imag = [q1(2); q1(3); q1(4)] ;
q2imag = [q2(2); q2(3); q2(4)];
qResultMag = q1(1)*q2(1) - dot(q1imag, q2imag);

qResultVect = q1(1)*q2imag + q2(1)*q1imag + cross(q1imag,q2imag);
qResult = [qResultMag; qResultVect];
end

== matlab function ame532Project1_GimbalDynamicsModel_2022b/Subsystem/Equations of Motion/Rotational Kinematics_Quaternions/quaternionToeuler ==
  data: qin input; yaw_deg output; pitch_deg output; roll_deg output
function [yaw_deg, pitch_deg, roll_deg] = quaternionsToEulerZYX(qin)
% Function to transfrom quaternion to Euler Angles in Tait-Bryan yaw,
% pitch, roll angle sequence

roll = atan2(2*(qin(1)*qin(2) + qin(3)*qin(4)), 1-2*(qin(2)^2 + qin(3)^2));
temp1 = sqrt(1+2*(qin(1)*qin(3)-qin(2)*qin(4)));
temp2 = sqrt(1-2*(qin(1)*qin(3) - qin(2)*qin(4)));
pitch = -pi/2 + 2*atan2(temp1, temp2);
yaw = atan2(2*(qin(1)*qin(4) + qin(2)*qin(3)) ,1-2*(qin(3)^2 + qin(4)^2));

yaw_deg = rad2deg(yaw);
pitch_deg = rad2deg(pitch);
roll_deg = rad2deg(roll);

end

== matlab function ame532Project1_GimbalDynamicsModel_2022b/Subsystem/Equations of Motion/Rotational Kinematics_Strapdown/Omega_B_N ==
  data: P_degPs input; y output; Q_degPs input; R_degPs input
function y = Omega_B_N(P_degPs,Q_degPs,R_degPs)
% Function used to generate cross product matrix of body rates (P,Q,R)
% w.r.t NED. This is basically a skew symmetric matrix
Omega_B_N = [0,-R_degPs,Q_degPs; R_degPs,0,-P_degPs; -Q_degPs,P_degPs,0];
y = Omega_B_N;

== matlab function ame532Project1_GimbalDynamicsModel_2022b/Subsystem/Equations of Motion/Rotational Kinematics_Strapdown/dcmTOeuler ==
  data: inputDCM input; yaw_deg output; pitch_deg output; roll_deg output
function [yaw_deg, pitch_deg, roll_deg] = dcmTOEuler_TB(inputDCM)
% This function takes in a dcm and outputs the euler angles in a Tait-Bryan
% ZYX angle sequence
c12 = inputDCM(1,2);
c11 = inputDCM(1,1);
c13 = inputDCM(1,3);
c23 = inputDCM(2,3);
c33 = inputDCM(3,3);
yaw_deg = atand(c12/c11);
pitch_deg = -asind(c13);
roll_deg = atand(c23/c33);
end

== matlab function ame532Project1_GimbalDynamicsModel_2022b/Subsystem/Equations of Motion/TransKin_RotKin_TansDynam/Rotational Kinematics_Euler/HinvMatrix ==
  data: pitchTheta input; hinv output; rollPhi input
function hinv = HinvMat(pitchTheta, rollPhi)
tThetasPhi = tan(pitchTheta) * sin(rollPhi);
tThetacPhi = tan(pitchTheta) * cos(rollPhi);
cPhi = cos(rollPhi);
sPhi = sin(rollPhi);
sPhiOvercTheta = sin(rollPhi)/cos(pitchTheta);
cPhiOvercTheta = cos(rollPhi)/cos(pitchTheta);

h = [1,tThetasPhi,tThetacPhi; 0,cPhi,-sPhi; 0,sPhiOvercTheta,cPhiOvercTheta];

hinv = h;

== matlab function ame532Project1_GimbalDynamicsModel_2022b/Subsystem/Equations of Motion/TransKin_RotKin_TansDynam/Rotational Kinematics_Quaternions/NormalizeQuaternion ==
  data: qin input; qoutNorm output
function qoutNorm = NormalizeQuaternion(qin)
qinMag = norm(qin);
qoutNorm = qin/qinMag;

== matlab function ame532Project1_GimbalDynamicsModel_2022b/Subsystem/Equations of Motion/TransKin_RotKin_TansDynam/Rotational Kinematics_Quaternions/quaternionMultiplication ==
  data: q1 input; qResult output; q2 input
function qResult = quaternionMultiplication(q1,q2)
q1imag = [q1(2); q1(3); q1(4)] ;
q2imag = [q2(2); q2(3); q2(4)];
qResultMag = q1(1)*q2(1) - dot(q1imag, q2imag);

qResultVect = q1(1)*q2imag + q2(1)*q1imag + cross(q1imag,q2imag);
qResult = [qResultMag; qResultVect];
end

== matlab function ame532Project1_GimbalDynamicsModel_2022b/Subsystem/Equations of Motion/TransKin_RotKin_TansDynam/Rotational Kinematics_Quaternions/quaternionToeuler ==
  data: qin input; yaw_deg output; pitch_deg output; roll_deg output
function [yaw_deg, pitch_deg, roll_deg] = quaternionsToEulerZYX(qin)
% Function to transfrom quaternion to Euler Angles in Tait-Bryan yaw,
% pitch, roll angle sequence

roll = atan2(2*(qin(1)*qin(2) + qin(3)*qin(4)), 1-2*(qin(2)^2 + qin(3)^2));
temp1 = sqrt(1+2*(qin(1)*qin(3)-qin(2)*qin(4)));
temp2 = sqrt(1-2*(qin(1)*qin(3) - qin(2)*qin(4)));
pitch = -pi/2 + 2*atan2(temp1, temp2);
yaw = atan2(2*(qin(1)*qin(4) + qin(2)*qin(3)) ,1-2*(qin(3)^2 + qin(4)^2));

yaw_deg = rad2deg(yaw);
pitch_deg = rad2deg(pitch);
roll_deg = rad2deg(roll);

end

== matlab function ame532Project1_GimbalDynamicsModel_2022b/Subsystem/Equations of Motion/TransKin_RotKin_TansDynam/Translational Kinematics/C_E_N ==
  data: lon_rad input; y output; lat_rad input
function y = NEDtoECEF(lon_rad, lat_rad)
% DCM to go from NED to ECEF frame

firstRot = [cos(lon_rad), cos(lon_rad), 0; -sin(lon_rad), cos(lon_rad), 0; 0, 0, 1;]; % Rotate about longitude first

secondRot = [0, 0, 1; 0, 1, 0; -1, 0,0]; % Left handed rotation of 90 deg 

thirdRot = [cos(lat_rad),0,sin(lat_rad); 0,1,0; -sin(lat_rad), 0, cos(lat_rad)];
% Multiply to get ECEF to NED DCM

c_NED_ECEF = thirdRot*secondRot*firstRot;
y = c_NED_ECEF';

== matlab function ame532Project1_GimbalDynamicsModel_2022b/Subsystem/Equations of Motion/TransKin_RotKin_TansDynam/Translational Kinematics/c_B_N ==
  data: yaw_rad input; outDCM output; pitch_rad input; roll_rad input
function outDCM = euler2DCM_TB(yaw_rad, pitch_rad, roll_rad)
% This functions takes in yaw, pitch and roll angles to compute the
% Tait-Bryan ZYX sequence DCM from reference frame (NED) to Body Frame
yawDCM = [cos(yaw_rad), sin(yaw_rad), 0; -sin(yaw_rad), cos(yaw_rad), 0; 0, 0, 1];
pitchDCM = [cos(pitch_rad), 0, -sin(pitch_rad); 0, 1, 0; sin(pitch_rad), 0, cos(pitch_rad)];

rollDCM = [1,0,0; 0, cos(roll_rad), sin(roll_rad); 0, -sin(roll_rad), cos(roll_rad)];
%outDCM = yawDCM*pitchDCM*rollDCM;
outDCM = rollDCM*pitchDCM*yawDCM;
end

== matlab function ame532Project1_GimbalDynamicsModel_2022b/Gimbal Aircraft dynamic sim/Rotational Kinematics/MATLAB Function5 ==
  data: DCM input; roll output; pitch output; yaw output
function [roll, pitch, yaw] = Euler_from_DCM(DCM)
   roll = atan2(DCM(2,3),DCM(3,3));
   pitch = asin(DCM(1,3));
   yaw = atan2(DCM(1,2),DCM(1,1));
end

== matlab function ame532Project1_GimbalDynamicsModel_2022b/Subsystem/Equations of Motion/TransKin_RotKin_TansDynam/Translational Kinematics/cartesianTOgeodetic ==
  data: cartVecPos input; lat_deg output; lon_deg output; r output
function [lat_deg, lon_deg, r]= cartesionTOgeodetic(cartVecPos)
% Cartesion coordinates must be w.r.t. ECEF frame
rEarth = 6378100; %m
r = norm(cartVecPos);
lat_deg = asind(cartVecPos(3)/r);
lon_deg = atan2d(cartVecPos(2),cartVecPos(1));

== matlab function ame532Project1_GimbalDynamicsModel_2022b/Subsystem/Equations of Motion/TransKin_RotKin_TansDynam/Translational Kinematics/C_EN from LAX to ECEF ==
  data: lat input; ZYXDCM output; long input
function ZYXDCM = DCM_from_Euler(lat,long) % sequence of rotation is lat long
%     yaw_matrix = [cos(yaw) sin(yaw) 0;
%                   -sin(yaw) cos(yaw) 0;
%                   0 0 1];
    lat_matrix = [cos(lat) 0 -sin(lat);
                    0           1           0;
                    sin(lat) 0  cos(lat)];
    long_matrix = [1            0           0;
                    0          cos(-long)    sin(-long);
                    0           -sin(-long)  cos(-long)];

    adjust_matrix = [cos(pi/2) 0 -sin(pi/2);
                    0           1           0;
                    sin(pi/2) 0  cos(pi/2)];
    ZYXDCM = adjust_matrix*long_matrix*lat_matrix;
end

%this rotational matrix turns lat long coordinate into a new C_EN
%assuming the N CS is lat and longitudinally rotated, then you would do
%-longditudinal rotation then lat rotation, then rotate 90 degrees again to
%match ECEF

== matlab function ame532Project1_GimbalDynamicsModel_2022b/Gimbal Aircraft dynamic sim/Rotational Kinematics/MATLAB Function6 ==
  data: DCM input; roll output; pitch output; yaw output
function [roll, pitch, yaw] = Euler_from_DCM(DCM)
   roll = atan2(DCM(2,3),DCM(3,3));
   pitch = -asin(DCM(1,3));
   yaw = atan2(DCM(1,2),DCM(1,1));
end

== matlab function ame532Project1_GimbalDynamicsModel_2022b/Gimbal Aircraft dynamic sim/Rotational Kinematics/MATLAB Function7 ==
  data: quat input; roll output; pitch output; yaw output
function [roll, pitch, yaw] = Euler_from_Quat(quat)
    DCM = zeros(3,3);
    DCM(1) = (quat(1)^2+quat(2)^2-quat(3)^2-quat(4)^2);
    DCM(2) = 2*(quat(2)*quat(3)-quat(1)*quat(4));
    DCM(3) = 2*(quat(2)*quat(4)+quat(1)*quat(3));
    DCM(4) = 2*(quat(2)*quat(3)+quat(1)*quat(4));
    DCM(5) = (quat(1)^2-quat(2)^2+quat(3)^2-quat(4)^2);
    DCM(6) = 2*(quat(3)*quat(4)-quat(1)*quat(2));
    DCM(7) = 2*(quat(2)*quat(4)-quat(1)*quat(3));
    DCM(8) = 2*(quat(3)*quat(4)+quat(1)*quat(2));
    DCM(9) = (quat(1)^2-quat(2)^2-quat(3)^2+quat(4)^2);

    roll = atan2(DCM(2,3),DCM(3,3));
    pitch = -asin(DCM(1,3));
    yaw = atan2(DCM(1,2),DCM(1,1));
end

== matlab function ame532Project1_GimbalDynamicsModel_2022b/Gimbal Aircraft dynamic sim/Rotational Kinematics/C_BN ==
  data: roll input; ZYXDCM output; pitch input; yaw input
function ZYXDCM = DCM_from_Euler(roll,pitch,yaw) % sequence is yaw pitch roll
    yaw_matrix = [cos(yaw) sin(yaw) 0;
                  -sin(yaw) cos(yaw) 0;
                  0 0 1];
    pitch_matrix = [cos(pitch) 0 -sin(pitch);
                    0           1           0;
                    sin(pitch) 0  cos(pitch)];
    roll_matrix = [1            0           0;
                    0          cos(roll)    sin(roll);
                    0           -sin(roll)  cos(roll)];
    ZYXDCM = roll_matrix*pitch_matrix*yaw_matrix;
end

== matlab function ame532Project1_GimbalDynamicsModel_2022b/Gimbal Aircraft dynamic sim/Rotational Kinematics/MATLAB Function8 ==
  data: roll input; ZYXquat_inv output; pitch input; yaw input; ZYXquat output
function [ZYXquat_inv,ZYXquat] = Quat_from_Euler(roll,pitch,yaw)
    q_yaw = zeros(4,1);
    q_yaw(1) = cos(yaw/2);
    q_yaw(2:4,1) = sin(yaw/2)*[0 0 1]';

    q_pitch = zeros(4,1);
    q_pitch(1) = cos(pitch/2);
    q_pitch(2:4,1) = sin(pitch/2)*[0 1 0]';

    q_roll = zeros(4,1);
    q_roll(1) = cos(roll/2);
    q_roll(2:4,1) = sin(roll/2)*[1 0 0]';
    
    inv_q_yaw = [q_yaw(1);-q_yaw(2:4)];
    inv_q_pitch = [q_pitch(1);-q_pitch(2:4)];
    inv_q_roll = [q_roll(1);-q_roll(2:4)];

    ZYXquat_inv = quat_mult(quat_mult(inv_q_roll,inv_q_pitch),inv_q_yaw);
    ZYXquat = quat_mult(quat_mult(q_yaw,q_pitch),q_roll);

end

function quat = quat_mult(q1,q2)
    quat = zeros(4,1);
    quat(1) = q1(1)*q2(1)-q1(2)*q2(2)-q1(3)*q2(3)-q1(4)*q2(4);
    quat(2) = q1(1)*q2(2)+q1(2)*q2(1)+q1(3)*q2(4)-q1(4)*q2(3);
    quat(3) = q1(1)*q2(3)-q1(2)*q2(4)+q1(3)*q2(1)+q1(4)*q2(2);
    quat(4) = q1(1)*q2(4)+q1(2)*q2(3)-q1(3)*q2(2)+q1(4)*q2(1);
end

== matlab function ame532Project1_GimbalDynamicsModel_2022b/Gimbal Aircraft dynamic sim/Rotational Kinematics/MATLAB Function9 ==
  data: q1 input; quat output; q2 input
function quat = quat_mult(q1,q2)
    quat = zeros(4,1);
    quat(1) = q1(1)*q2(1)-q1(2)*q2(2)-q1(3)*q2(3)-q1(4)*q2(4);
    quat(2) = q1(1)*q2(2)+q1(2)*q2(1)+q1(3)*q2(4)-q1(4)*q2(3);
    quat(3) = q1(1)*q2(3)-q1(2)*q2(4)+q1(3)*q2(1)+q1(4)*q2(2);
    quat(4) = q1(1)*q2(4)+q1(2)*q2(3)-q1(3)*q2(2)+q1(4)*q2(1);
end

== matlab function ame532Project1_GimbalDynamicsModel_2022b/Gimbal Aircraft dynamic sim/Unused tranlational kinmatics/C_EN4 ==
  data: roll input; ZYXDCM output; pitch input; yaw input
function ZYXDCM = DCM_from_Euler(roll,pitch,yaw) % sequence is yaw pitch roll
    yaw_matrix = [cos(yaw) sin(yaw) 0;
                  -sin(yaw) cos(yaw) 0;
                  0 0 1];
    pitch_matrix = [cos(pitch) 0 -sin(pitch);
                    0           1           0;
                    sin(pitch) 0  cos(pitch)];
    roll_matrix = [1            0           0;
                    0          cos(roll)    sin(roll);
                    0           -sin(roll)  cos(roll)];
    ZYXDCM = roll_matrix*pitch_matrix*yaw_matrix;
end

== matlab function ame532Project1_GimbalDynamicsModel_2022b/Gimbal Aircraft dynamic sim/translational dynamics/MATLAB Function10 ==
  data: p input; Cross_Product_Matrix output; q input; r input
function Cross_Product_Matrix = omega_to_cross_product_matrix(p,q,r)

    Cross_Product_Matrix =[0 -r q; r 0 -p; -q p 0];

end

== matlab function ame532Project1_GimbalDynamicsModel_2022b/Gimbal Aircraft dynamic sim/aeroforce coefficient block/MATLAB Function ==
  data: AR_matrix input; CL_a output
function CL_a = Calculate_CL_a(AR_matrix)

CL_a = zeros(4,1);

for i = 1:4
    CL_a(i) = 2*pi*(AR_matrix(i)/(2+AR_matrix(i)));
end

== matlab function ame532Project1_GimbalDynamicsModel_2022b/Gimbal Aircraft dynamic sim/Translational Kinematics/new C_EN base on cart. coordinate1 ==
  data: lat input; ZYXDCM output; long input
function ZYXDCM = DCM_from_Euler(lat,long) % sequence of rotation is lat long
%     yaw_matrix = [cos(yaw) sin(yaw) 0;
%                   -sin(yaw) cos(yaw) 0;
%                   0 0 1];
    lat_matrix = [cos(lat) 0 -sin(lat);
                    0           1           0;
                    sin(lat) 0  cos(lat)];
    long_matrix = [1            0           0;
                    0          cos(-long)    sin(-long);
                    0           -sin(-long)  cos(-long)];

    adjust_matrix = [cos(pi/2) 0 -sin(pi/2);
                    0           1           0;
                    sin(pi/2) 0  cos(pi/2)];
    ZYXDCM = adjust_matrix*long_matrix*lat_matrix;
end

%this rotational matrix turns lat long coordinate into a new C_EN
%assuming the N CS is lat and longitudinally rotated, then you would do
%-longditudinal rotation then lat rotation, then rotate 90 degrees again to
%match ECEF

== matlab function ame532Project1_GimbalDynamicsModel_2022b/Gimbal Aircraft dynamic sim/measurement subsystem/MATLAB Function ==
  data: velocity input; magnitude output
function magnitude = magnitude_from_vector(velocity)

magnitude = sqrt(velocity(1)^2+velocity(2)^2+velocity(3)^2);

end

== matlab function ame532Project1_GimbalDynamicsModel_2022b/Gimbal Aircraft dynamic sim/mass & aero property calculation/CG calculation ==
  data: M_matrix input; cg_x output; cg_y output; cg_z output
function [cg_x, cg_y, cg_z] = CG_calc(M_matrix)

mass_col = M_matrix(:,1);
x_col = M_matrix(:,5);
y_col = M_matrix(:,6);
z_col = M_matrix(:,7);

cg_x = sum(mass_col.*x_col)/(sum(mass_col));
cg_y = sum(mass_col.*y_col)/(sum(mass_col));
cg_z = sum(mass_col.*z_col)/(sum(mass_col));

end

== matlab function ame532Project1_GimbalDynamicsModel_2022b/Gimbal Aircraft dynamic sim/mass & aero property calculation/MATLAB Function ==
  data: cg_location input; M_matrix input; J_matrix output
function J_matrix = fcn(cg_location,M_matrix)


mass_col = M_matrix(:,1);
x_dim = M_matrix(:,2);
y_dim = M_matrix(:,3);
z_dim = M_matrix(:,4);
x_loc = M_matrix(:,5);
y_loc = M_matrix(:,6);
z_loc = M_matrix(:,7);

Ixx = zeros(11,1);
Iyy = zeros(11,1);
Izz = zeros(11,1);
Ixz = zeros(11,1);
Izx = Ixz;
Ixy = zeros(11,1);
Iyx = Ixy;
Iyz = zeros(11,1);
Izy = Iyz;

J_matrix = zeros(3,3);

% all moment of inertial is calculated wrt to CG

for i = 1:11
    Ixx(i) = mass_col(i)*(y_dim(i)^2+z_dim(i)^2)/(12)+mass_col(i)*((y_loc(i)-cg_location(2))^2+(z_loc(i)-cg_location(3))^2); % check discussion post
    Iyy(i) = mass_col(i)*(x_dim(i)^2+z_dim(i)^2)/(12)+mass_col(i)*((x_loc(i)-cg_location(1))^2+(z_loc(i)-cg_location(3))^2);
    Izz(i) = mass_col(i)*(y_dim(i)^2+x_dim(i)^2)/(12)+mass_col(i)*((y_loc(i)-cg_location(2))^2+(x_loc(i)-cg_location(1))^2);
    Ixz(i) = mass_col(i)*((z_loc(i)-cg_location(3))*(x_loc(i)-cg_location(1)));
    Ixy(i) = mass_col(i)*((x_loc(i)-cg_location(1))*(y_loc(i)-cg_location(2)));
    Iyz(i) = mass_col(i)*((y_loc(i)-cg_location(2))*(z_loc(i)-cg_location(3)));


end

J_matrix(1,1) = sum(Ixx);
J_matrix(2,2) = sum(Iyy);
J_matrix(3,3) = sum(Izz);
J_matrix(1,2) = sum(Ixy);
J_matrix(2,1) = sum(Ixy);
J_matrix(1,3) = sum(Ixz);
J_matrix(3,1) = sum(Ixz);
J_matrix(2,3) = sum(Iyz);
J_matrix(3,2) = sum(Iyz);

J_matrix = J_matrix./1000;
end

== matlab function ame532Project1_GimbalDynamicsModel_2022b/Gimbal Aircraft dynamic sim/Translational Kinematics/C_EN from LAX to ECEF ==
  data: lat input; ZYXDCM output; long input
function ZYXDCM = DCM_from_Euler(lat,long) % sequence of rotation is lat long
%     yaw_matrix = [cos(yaw) sin(yaw) 0;
%                   -sin(yaw) cos(yaw) 0;
%                   0 0 1];
    lat_matrix = [cos(lat) 0 -sin(lat);
                    0           1           0;
                    sin(lat) 0  cos(lat)];
    long_matrix = [1            0           0;
                    0          cos(-long)    sin(-long);
                    0           -sin(-long)  cos(-long)];

    adjust_matrix = [cos(pi/2) 0 -sin(pi/2);
                    0           1           0;
                    sin(pi/2) 0  cos(pi/2)];
    ZYXDCM = adjust_matrix*long_matrix*lat_matrix;
end

%this rotational matrix turns lat long coordinate into a new C_EN
%assuming the N CS is lat and longitudinally rotated, then you would do
%-longditudinal rotation then lat rotation, then rotate 90 degrees again to
%match ECEF

== matlab function ame532Project1_GimbalDynamicsModel_2022b/Gimbal Aircraft dynamic sim/mass & aero property calculation/MATLAB Function2 ==
  data: M_matrix input; aero_prop output
function aero_prop = fcn(M_matrix)

aero_prop = zeros(4,7);
for i = 1:4
    aero_prop(i,1:3) = M_matrix(i,5:7);
    aero_prop(i,4) = M_matrix(i,2);
end

%% define span for each surface

    aero_prop(1,5) = M_matrix(1,3); %right wing
    aero_prop(2,5) = M_matrix(2,3); %left wing
    aero_prop(3,5) = M_matrix(3,3); %hor stab.
    aero_prop(4,5) = M_matrix(4,4); %ver stab.
%% define area and aspect ratio for each surface

for i = 1:4
    aero_prop(i,6) = aero_prop(i,4)*aero_prop(i,5);
    aero_prop(i,7) = aero_prop(i,5)/aero_prop(i,4);
end

== matlab function ame532Project1_GimbalDynamicsModel_2022b/Gimbal Aircraft dynamic sim/aeroforce coefficient block/extract matrix function ==
  data: aero_surface_matrix input; AR_matrix output
function AR_matrix = Extract_AR(aero_surface_matrix)

AR_matrix = aero_surface_matrix(:,7);
end

== matlab function ame532Project1_GimbalDynamicsModel_2022b/Gimbal Aircraft dynamic sim/aeroforce coefficient block/calculatie alpha ==
  data: i0 input; alpha output; v_B input; n_vector input; wind_w input; v_B_BA output; C_BN input
function [alpha,v_B_BA] = fcn(i0,v_B,n_vector,wind_w,C_BN)

alpha = zeros(4,1);
% this function calculates alpha that the aero surface sees

v_B_BA = v_B - C_BN*wind_w;

for i = 1:4
    alpha(i) = i0(i) - asin(dot(v_B_BA,n_vector(:,i))/norm(v_B_BA));
end

== matlab function ame532Project1_GimbalDynamicsModel_2022b/Gimbal Aircraft dynamic sim/aeroforce coefficient block/MATLAB Function1 ==
  data: CL0 input; CL_s output; CL_a input; alpha input
function CL_s = calculate_CL_s(CL0,CL_a,alpha)

CL_s = zeros(4,1);

for i = 1:4
    CL_s(i) = CL0(i)+CL_a(i)*alpha(i);
end

== matlab function ame532Project1_GimbalDynamicsModel_2022b/Gimbal Aircraft dynamic sim/aeroforce coefficient block/MATLAB Function2 ==
  data: CD_0 input; CD_a input; CD_s output; alpha_0 input; alpha input; CL_s input; e input; AR input
function CD_s = calculate_CD_s(CD_0,CD_a,alpha_0,alpha,CL_s,e,AR)
CD_s = zeros(4,1);

for i = 1:4
    
    CD_s(i) = CD_0(i) + CD_a(i)*(alpha(i)-alpha_0(i))^2+(CL_s(i)^2)/(pi*e(i)*AR(i));

end

== matlab function ame532Project1_GimbalDynamicsModel_2022b/Gimbal Aircraft dynamic sim/aeroforce coefficient block/extract matrix function1 ==
  data: aero_surface_matrix input; AR_matrix output
function AR_matrix = Extract_AR(aero_surface_matrix)

AR_matrix = aero_surface_matrix(:,7);
end
